simulink model "sampleModel2438_pp"  (R2018a)
settings: Solver=VariableStepAuto  StartTime=0.0  StopTime=10.0  RelTol=1e-3
undefined symbols (not defined in the file or in its folder): DiscIntNeverNeededParam, sigbuilder_block
libraries: simulink x299
(part 4 of 6)

== system sampleModel2438_pp/cfblk261 ==
  cfblk1 : Inport
  Action Port : ActionPort  ActionType=else
  cfblk10 : DiscreteIntegrator  SampleTime=-1  ICPrevOutput=DiscIntNeverNeededParam  ICPrevScaledInput=DiscIntNeverNeededParam
  cfblk12 : Delay
  cfblk3 : DiscreteFir
  cfblk4 : DiscreteFilter
  cfblk5 : UnitDelay  SampleTime=-1
  cfblk6 : simulink/Discrete/Transfer Fcn Real Zero  ZeroZ=0.75  ICPrevInput=0.0  DoSatur=off
      settings: SourceProductName=Simulink  SourceProductBaseCode=SL
  cfblk7 : DiscreteFilter
  cfblk8 : simulink/Continuous/PID Controller (2DOF)  Controller=PID  TimeDomain=Discrete-time  SampleTime=-1  IntegratorMethod=Forward Euler  FilterMethod=Forward Euler  Form=Parallel  UseFilter=on  ControllerParametersSource=internal  P=1  I=1  D=0  N=100  b=1  c=1  InitialConditionSource=internal  InitialConditionForIntegrator=0  InitialConditionForFilter=0  ExternalReset=none  LimitOutput=off  UpperSaturationLimit=inf  LowerSaturationLimit=-inf  LinearizeAsGain=off  AntiWindupMode=none  Kb=1  TrackingMode=off  Kt=1  PParamMin=[]  PParamMax=[]  IParamMin=[]  IParamMax=[]  DParamMin=[]  DParamMax=[]  NParamMin=[]  NParamMax=[]  bParamMin=[]  bParamMax=[]  cParamMin=[]  cParamMax=[]  KbParamMin=[]  KbParamMax=[]  KtParamMin=[]  KtParamMax=[]  POutMin=[]  POutMax=[]  IOutMin=[]  IOutMax=[]  DOutMin=[]  DOutMax=[]  NOutMin=[]  NOutMax=[]  bOutMin=[]  bOutMax=[]  cOutMin=[]  cOutMax=[]  KbOutMin=[]  KbOutMax=[]  KtOutMin=[]  KtOutMax=[]  IntegratorOutMin=[]  IntegratorOutMax=[]  FilterOutMin=[]  FilterOutMax=[]  SumOutMin=[]  SumOutMax=[]  Sum1OutMin=[]  Sum1OutMax=[]  Sum2OutMin=[]  Sum2OutMax=[]  Sum3OutMin=[]  Sum3OutMax=[]  SumI1OutMin=[]  SumI1OutMax=[]  SumI2OutMin=[]  SumI2OutMax=[]  SumI3OutMin=[]  SumI3OutMax=[]  SumDOutMin=[]  SumDOutMax=[]  SaturationOutMin=[]  SaturationOutMax=[]  IntegratorContinuousStateAttributes=''  IntegratorStateMustResolveToSignalObject=off  IntegratorRTWStateStorageClass=Auto  FilterContinuousStateAttributes=''  FilterStateMustResolveToSignalObject=off  FilterRTWStateStorageClass=Auto  DifferentiatorICPrevScaledInput=0  DifferentiatorOutMin=[]  DifferentiatorOutMax=[]  FilterDiffOutCoefMin=[]  FilterDiffOutCoefMax=[]  SumDenOutMin=[]  SumDenOutMax=[]  SumNumOutMin=[]  SumNumOutMax=[]  ReciprocalOutMin=[]  ReciprocalOutMax=[]  DivideOutMin=[]  DivideOutMax=[]  TunerSelectOption=Transfer Function Based (PID Tuner App)
  cfblk9 : DiscreteZeroPole  Poles=[0 0.5]  Gain=1  SampleTime=-1
  cyemi_{797..806} (10 alike) : DataTypeConversion  OutDataTypeStr=double
  cfblk2 : Outport
  cfblk11 : Outport  Port=2
  wires:
  cfblk5/1 -> cyemi_803/1, cyemi_806/1
  cfblk7/1 -> cfblk2/1
  cfblk1/1 -> cyemi_801/1, cyemi_804/1
  cfblk3/1 -> cfblk11/1
  cyemi_797/1 -> cfblk10/1
  cfblk6/1 -> cyemi_797/1
  cyemi_798/1 -> cfblk12/1
  cfblk10/1 -> cyemi_798/1
  cyemi_799/1 -> cfblk3/1
  cfblk4/1 -> cyemi_799/1
  cyemi_800/1 -> cfblk4/1
  cfblk9/1 -> cyemi_800/1
  cyemi_801/1 -> cfblk5/1
  cyemi_802/1 -> cfblk6/1
  cfblk8/1 -> cyemi_802/1
  cyemi_803/1 -> cfblk7/1
  cyemi_804/1 -> cfblk8/1
  cyemi_805/1 -> cfblk8/2
  cfblk12/1 -> cyemi_805/1
  cyemi_806/1 -> cfblk9/1

== system sampleModel2438_pp/cfblk262 ==
  cfblk1 : Inport
  Action Port : ActionPort  ActionType=then
  cfblk10 : Delay
  cfblk11 : Delay
  cfblk12 : Delay
  cfblk3 : simulink/Discrete/Transfer Fcn First Order  PoleZ=0.95  ICPrevOutput=0.0  DoSatur=off
      settings: SourceProductName=Simulink
  cfblk4 : simulink/Discrete/Transfer Fcn First Order  PoleZ=0.95  ICPrevOutput=0.0  DoSatur=off
      settings: SourceProductName=Simulink
  cfblk5 : simulink/Discrete/Transfer Fcn First Order  PoleZ=0.95  ICPrevOutput=0.0  DoSatur=off
      settings: SourceProductName=Simulink
  cfblk6 : If  SampleTime=1
  cfblk8 : Subsystem  TreatAsAtomicUnit=on
  cfblk9 : Subsystem  TreatAsAtomicUnit=on
  cyemi_{808..817,836..839} (14 alike) : DataTypeConversion  OutDataTypeStr=double
  cfblk2 : Outport
  cfblk7 : Outport  Port=2
  wires:
  cfblk9/1(cfblk2) -> cfblk7/1
  cfblk1/1 -> cyemi_813/1, cyemi_836/1
  cfblk3/1 -> cyemi_809/1, cyemi_810/1
  cfblk4/1 -> cfblk2/1, cyemi_808/1
  cfblk5/1 -> cyemi_814/1, cyemi_815/1, cyemi_838/1
  cfblk9/2(cfblk14) -> cyemi_812/1, cyemi_816/1
  cfblk6/1 -> cfblk8/Action
  cfblk6/2 -> cfblk9/Action
  cyemi_808/1 -> cfblk10/1
  cyemi_809/1 -> cfblk11/1
  cyemi_810/1 -> cfblk12/1
  cyemi_811/1 -> cfblk3/1
  cfblk8/1(cfblk2) -> cyemi_811/1
  cyemi_812/1 -> cfblk4/1
  cyemi_813/1 -> cfblk5/1
  cyemi_814/1 -> cfblk6/1
  cyemi_815/1 -> cfblk8/1(cfblk1)
  cyemi_816/1 -> cfblk8/2(cfblk14)
  cyemi_817/1 -> cfblk8/3(cfblk15)
  cfblk12/1 -> cyemi_817/1
  cyemi_836/1 -> cfblk9/1(cfblk1)
  cyemi_837/1 -> cfblk9/2(cfblk11)
  cfblk11/1 -> cyemi_837/1
  cyemi_838/1 -> cfblk9/3(cfblk12)
  cyemi_839/1 -> cfblk9/4(cfblk13)
  cfblk10/1 -> cyemi_839/1

== system sampleModel2438_pp/cfblk263 ==
  cfblk1 : Inport
  cfblk5 : Inport  Port=2
  cfblk6 : Inport  Port=3
  cfblk7 : Inport  Port=4
  Action Port : ActionPort  ActionType=else
  cfblk10 : Delay
  cfblk3 : Delay  ShowEnablePort=on
      settings: InputPortMap=u0,e6
  cfblk4 : Delay
  cyemi_{855..858} (4 alike) : DataTypeConversion  OutDataTypeStr=double
  cfblk2 : Outport
  cfblk8 : Outport  Port=2
  cfblk9 : Outport  Port=3
  wires:
  cfblk1/1 -> cfblk2/1
  cfblk6/1 -> cfblk9/1
  cfblk7/1 -> cfblk8/1
  cyemi_855/1 -> cfblk10/1
  cfblk4/1 -> cyemi_855/1
  cyemi_856/1 -> cfblk3/1
  cfblk5/1 -> cyemi_856/1
  cyemi_857/1 -> cfblk3/2
  cfblk10/1 -> cyemi_857/1
  cyemi_858/1 -> cfblk4/1
  cfblk3/1 -> cyemi_858/1

== system sampleModel2438_pp/cfblk264 ==
  cfblk1 : Inport
  cfblk6 : Inport  Port=2
  cfblk7 : Inport  Port=3
  Action Port : ActionPort  ActionType=then
  cfblk3 : simulink/Discrete/Tapped Delay  vinit=0.0  samptime=-1  NumDelays=1  DelayOrder=Oldest  includeCurrent=off
  cfblk4 : UnitDelay  SampleTime=-1
  cfblk5 : simulink/Discrete/Transfer Fcn Real Zero  ZeroZ=0.75  ICPrevInput=0.0  DoSatur=off
      settings: SourceProductName=Simulink  SourceProductBaseCode=SL
  cyemi_862 : DataTypeConversion  OutDataTypeStr=double
  cyemi_863 : DataTypeConversion  OutDataTypeStr=double
  cyemi_864 : DataTypeConversion  OutDataTypeStr=double
  cfblk2 : Outport
  wires:
  cfblk1/1 -> cfblk2/1
  cyemi_862/1 -> cfblk3/1
  cfblk7/1 -> cyemi_862/1
  cyemi_863/1 -> cfblk4/1
  cfblk5/1 -> cyemi_863/1
  cyemi_864/1 -> cfblk5/1
  cfblk3/1 -> cyemi_864/1

== system sampleModel2438_pp/cfblk265 ==
  cfblk1 : Inport
  cfblk6 : Inport  Port=2
  cfblk7 : Inport  Port=3
  cfblk8 : Inport  Port=4
  cfblk9 : Inport  Port=5
  Action Port : ActionPort  ActionType=else
  cfblk3 : DiscreteTransferFcn
  cfblk4 : DiscreteTransferFcn
  cfblk5 : DiscreteStateSpace  SampleTime=-1
  cyemi_870 : DataTypeConversion  OutDataTypeStr=double
  cyemi_871 : DataTypeConversion  OutDataTypeStr=double
  cyemi_872 : DataTypeConversion  OutDataTypeStr=double
  cfblk2 : Outport
  cfblk10 : Outport  Port=2
  wires:
  cfblk5/1 -> cfblk2/1
  cfblk9/1 -> cfblk10/1
  cyemi_870/1 -> cfblk3/1
  cfblk1/1 -> cyemi_870/1
  cyemi_871/1 -> cfblk4/1
  cfblk6/1 -> cyemi_871/1
  cyemi_872/1 -> cfblk5/1
  cfblk4/1 -> cyemi_872/1

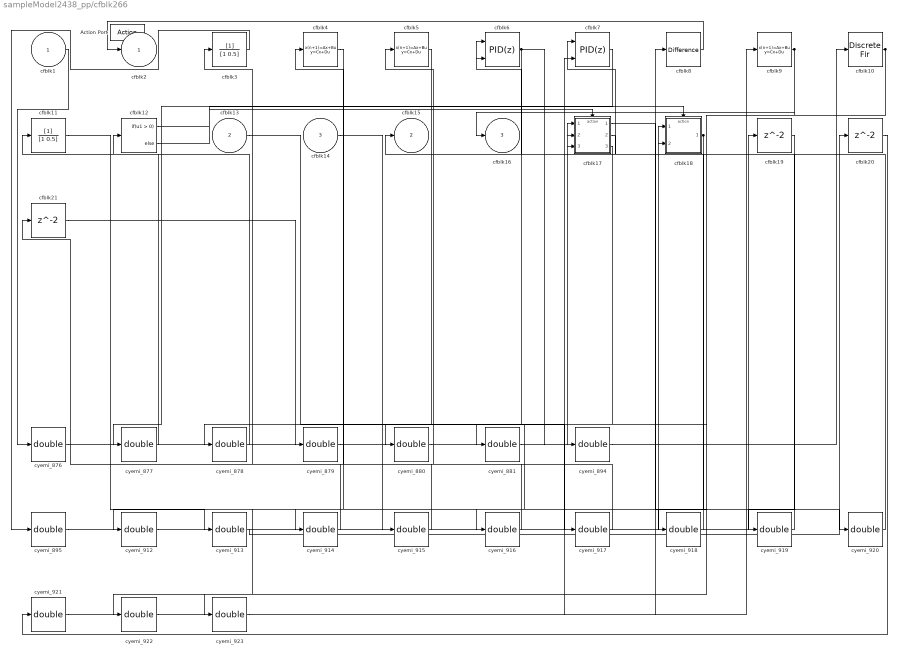
== system sampleModel2438_pp/cfblk266 ==
  cfblk1 : Inport
  cfblk13 : Inport  Port=2
  cfblk14 : Inport  Port=3
  Action Port : ActionPort  ActionType=then
  cfblk10 : DiscreteFir
  cfblk11 : DiscreteFilter
  cfblk12 : If  SampleTime=1
  cfblk17 : Subsystem  TreatAsAtomicUnit=on
  cfblk18 : Subsystem  TreatAsAtomicUnit=on
  cfblk19 : Delay
  cfblk20 : Delay
  cfblk21 : Delay
  cfblk3 : DiscreteFilter
  cfblk4 : DiscreteStateSpace  SampleTime=-1
  cfblk5 : DiscreteStateSpace  SampleTime=-1
  cfblk6 : simulink/Continuous/PID Controller (2DOF)  Controller=PID  TimeDomain=Discrete-time  SampleTime=-1  IntegratorMethod=Forward Euler  FilterMethod=Forward Euler  Form=Parallel  UseFilter=on  ControllerParametersSource=internal  P=1  I=1  D=0  N=100  b=1  c=1  InitialConditionSource=internal  InitialConditionForIntegrator=0  InitialConditionForFilter=0  ExternalReset=none  LimitOutput=off  UpperSaturationLimit=inf  LowerSaturationLimit=-inf  LinearizeAsGain=off  AntiWindupMode=none  Kb=1  TrackingMode=off  Kt=1  PParamMin=[]  PParamMax=[]  IParamMin=[]  IParamMax=[]  DParamMin=[]  DParamMax=[]  NParamMin=[]  NParamMax=[]  bParamMin=[]  bParamMax=[]  cParamMin=[]  cParamMax=[]  KbParamMin=[]  KbParamMax=[]  KtParamMin=[]  KtParamMax=[]  POutMin=[]  POutMax=[]  IOutMin=[]  IOutMax=[]  DOutMin=[]  DOutMax=[]  NOutMin=[]  NOutMax=[]  bOutMin=[]  bOutMax=[]  cOutMin=[]  cOutMax=[]  KbOutMin=[]  KbOutMax=[]  KtOutMin=[]  KtOutMax=[]  IntegratorOutMin=[]  IntegratorOutMax=[]  FilterOutMin=[]  FilterOutMax=[]  SumOutMin=[]  SumOutMax=[]  Sum1OutMin=[]  Sum1OutMax=[]  Sum2OutMin=[]  Sum2OutMax=[]  Sum3OutMin=[]  Sum3OutMax=[]  SumI1OutMin=[]  SumI1OutMax=[]  SumI2OutMin=[]  SumI2OutMax=[]  SumI3OutMin=[]  SumI3OutMax=[]  SumDOutMin=[]  SumDOutMax=[]  SaturationOutMin=[]  SaturationOutMax=[]  IntegratorContinuousStateAttributes=''  IntegratorStateMustResolveToSignalObject=off  IntegratorRTWStateStorageClass=Auto  FilterContinuousStateAttributes=''  FilterStateMustResolveToSignalObject=off  FilterRTWStateStorageClass=Auto  DifferentiatorICPrevScaledInput=0  DifferentiatorOutMin=[]  DifferentiatorOutMax=[]  FilterDiffOutCoefMin=[]  FilterDiffOutCoefMax=[]  SumDenOutMin=[]  SumDenOutMax=[]  SumNumOutMin=[]  SumNumOutMax=[]  ReciprocalOutMin=[]  ReciprocalOutMax=[]  DivideOutMin=[]  DivideOutMax=[]  TunerSelectOption=Transfer Function Based (PID Tuner App)
  cfblk7 : simulink/Continuous/PID Controller (2DOF)  Controller=PID  TimeDomain=Discrete-time  SampleTime=-1  IntegratorMethod=Forward Euler  FilterMethod=Forward Euler  Form=Parallel  UseFilter=on  ControllerParametersSource=internal  P=1  I=1  D=0  N=100  b=1  c=1  InitialConditionSource=internal  InitialConditionForIntegrator=0  InitialConditionForFilter=0  ExternalReset=none  LimitOutput=off  UpperSaturationLimit=inf  LowerSaturationLimit=-inf  LinearizeAsGain=off  AntiWindupMode=none  Kb=1  TrackingMode=off  Kt=1  PParamMin=[]  PParamMax=[]  IParamMin=[]  IParamMax=[]  DParamMin=[]  DParamMax=[]  NParamMin=[]  NParamMax=[]  bParamMin=[]  bParamMax=[]  cParamMin=[]  cParamMax=[]  KbParamMin=[]  KbParamMax=[]  KtParamMin=[]  KtParamMax=[]  POutMin=[]  POutMax=[]  IOutMin=[]  IOutMax=[]  DOutMin=[]  DOutMax=[]  NOutMin=[]  NOutMax=[]  bOutMin=[]  bOutMax=[]  cOutMin=[]  cOutMax=[]  KbOutMin=[]  KbOutMax=[]  KtOutMin=[]  KtOutMax=[]  IntegratorOutMin=[]  IntegratorOutMax=[]  FilterOutMin=[]  FilterOutMax=[]  SumOutMin=[]  SumOutMax=[]  Sum1OutMin=[]  Sum1OutMax=[]  Sum2OutMin=[]  Sum2OutMax=[]  Sum3OutMin=[]  Sum3OutMax=[]  SumI1OutMin=[]  SumI1OutMax=[]  SumI2OutMin=[]  SumI2OutMax=[]  SumI3OutMin=[]  SumI3OutMax=[]  SumDOutMin=[]  SumDOutMax=[]  SaturationOutMin=[]  SaturationOutMax=[]  IntegratorContinuousStateAttributes=''  IntegratorStateMustResolveToSignalObject=off  IntegratorRTWStateStorageClass=Auto  FilterContinuousStateAttributes=''  FilterStateMustResolveToSignalObject=off  FilterRTWStateStorageClass=Auto  DifferentiatorICPrevScaledInput=0  DifferentiatorOutMin=[]  DifferentiatorOutMax=[]  FilterDiffOutCoefMin=[]  FilterDiffOutCoefMax=[]  SumDenOutMin=[]  SumDenOutMax=[]  SumNumOutMin=[]  SumNumOutMax=[]  ReciprocalOutMin=[]  ReciprocalOutMax=[]  DivideOutMin=[]  DivideOutMax=[]  TunerSelectOption=Transfer Function Based (PID Tuner App)
  cfblk8 : simulink/Discrete/Difference  ICPrevInput=0.0  OutMin=[]  OutMax=[]  OutDataTypeStr=Inherit: Inherit via back propagation  OutDataType=fixdt(1, 16)  OutScaling=2^-10  DoSatur=off
  cfblk9 : DiscreteStateSpace  SampleTime=-1
  cyemi_{876..881,894..895,912..923} (20 alike) : DataTypeConversion  OutDataTypeStr=double
  cfblk2 : Outport
  cfblk15 : Outport  Port=2
  cfblk16 : Outport  Port=3
  wires:
  cfblk6/1 -> cyemi_880/1, cyemi_894/1
  cfblk17/2(cfblk11) -> cfblk15/1
  cfblk8/1 -> cfblk2/1
  cfblk10/1 -> cyemi_881/1, cyemi_918/1
  cfblk18/1(cfblk2) -> cyemi_912/1, cyemi_923/1
  cfblk9/1 -> cfblk16/1, cyemi_922/1
  cfblk12/1 -> cfblk17/Action
  cfblk12/2 -> cfblk18/Action
  cyemi_876/1 -> cfblk10/1
  cfblk1/1 -> cyemi_876/1
  cyemi_877/1 -> cfblk11/1
  cfblk7/1 -> cyemi_877/1
  cyemi_878/1 -> cfblk12/1
  cfblk5/1 -> cyemi_878/1
  cyemi_879/1 -> cfblk17/1(cfblk1)
  cfblk21/1 -> cyemi_879/1
  cyemi_880/1 -> cfblk17/2(cfblk9)
  cyemi_881/1 -> cfblk17/3(cfblk10)
  cyemi_894/1 -> cfblk18/1(cfblk1)
  cyemi_895/1 -> cfblk18/2(cfblk14)
  cfblk3/1 -> cyemi_895/1
  cyemi_912/1 -> cfblk19/1
  cyemi_913/1 -> cfblk20/1
  cfblk11/1 -> cyemi_913/1
  cyemi_914/1 -> cfblk21/1
  cfblk4/1 -> cyemi_914/1
  cyemi_915/1 -> cfblk3/1
  cfblk14/1 -> cyemi_915/1
  cyemi_916/1 -> cfblk4/1
  cfblk17/3(cfblk12) -> cyemi_916/1
  cyemi_917/1 -> cfblk5/1
  cfblk13/1 -> cyemi_917/1
  cyemi_918/1 -> cfblk6/1
  cyemi_919/1 -> cfblk6/2
  cfblk19/1 -> cyemi_919/1
  cyemi_920/1 -> cfblk7/1
  cfblk17/1(cfblk2) -> cyemi_920/1
  cyemi_921/1 -> cfblk7/2
  cfblk20/1 -> cyemi_921/1
  cyemi_922/1 -> cfblk8/1
  cyemi_923/1 -> cfblk9/1

== system sampleModel2438_pp/cfblk267 ==
  cfblk1 : Inport
  cfblk10 : Inport  Port=2
  cfblk11 : Inport  Port=3
  cfblk12 : Inport  Port=4
  Action Port : ActionPort  ActionType=else
  cfblk15 : Delay
  cfblk3 : simulink/Discrete/Difference  ICPrevInput=0.0  OutMin=[]  OutMax=[]  OutDataTypeStr=Inherit: Inherit via back propagation  OutDataType=fixdt(1, 16)  OutScaling=2^-10  DoSatur=off
  cfblk4 : DiscreteTransferFcn
  cfblk5 : simulink/Discrete/Transfer Fcn Real Zero  ZeroZ=0.75  ICPrevInput=0.0  DoSatur=off
      settings: SourceProductName=Simulink  SourceProductBaseCode=SL
  cfblk6 : DiscreteIntegrator  SampleTime=-1  ICPrevOutput=DiscIntNeverNeededParam  ICPrevScaledInput=DiscIntNeverNeededParam
  cfblk7 : simulink/Continuous/PID Controller (2DOF)  Controller=PID  TimeDomain=Discrete-time  SampleTime=-1  IntegratorMethod=Forward Euler  FilterMethod=Forward Euler  Form=Parallel  UseFilter=on  ControllerParametersSource=internal  P=1  I=1  D=0  N=100  b=1  c=1  InitialConditionSource=internal  InitialConditionForIntegrator=0  InitialConditionForFilter=0  ExternalReset=none  LimitOutput=off  UpperSaturationLimit=inf  LowerSaturationLimit=-inf  LinearizeAsGain=off  AntiWindupMode=none  Kb=1  TrackingMode=off  Kt=1  PParamMin=[]  PParamMax=[]  IParamMin=[]  IParamMax=[]  DParamMin=[]  DParamMax=[]  NParamMin=[]  NParamMax=[]  bParamMin=[]  bParamMax=[]  cParamMin=[]  cParamMax=[]  KbParamMin=[]  KbParamMax=[]  KtParamMin=[]  KtParamMax=[]  POutMin=[]  POutMax=[]  IOutMin=[]  IOutMax=[]  DOutMin=[]  DOutMax=[]  NOutMin=[]  NOutMax=[]  bOutMin=[]  bOutMax=[]  cOutMin=[]  cOutMax=[]  KbOutMin=[]  KbOutMax=[]  KtOutMin=[]  KtOutMax=[]  IntegratorOutMin=[]  IntegratorOutMax=[]  FilterOutMin=[]  FilterOutMax=[]  SumOutMin=[]  SumOutMax=[]  Sum1OutMin=[]  Sum1OutMax=[]  Sum2OutMin=[]  Sum2OutMax=[]  Sum3OutMin=[]  Sum3OutMax=[]  SumI1OutMin=[]  SumI1OutMax=[]  SumI2OutMin=[]  SumI2OutMax=[]  SumI3OutMin=[]  SumI3OutMax=[]  SumDOutMin=[]  SumDOutMax=[]  SaturationOutMin=[]  SaturationOutMax=[]  IntegratorContinuousStateAttributes=''  IntegratorStateMustResolveToSignalObject=off  IntegratorRTWStateStorageClass=Auto  FilterContinuousStateAttributes=''  FilterStateMustResolveToSignalObject=off  FilterRTWStateStorageClass=Auto  DifferentiatorICPrevScaledInput=0  DifferentiatorOutMin=[]  DifferentiatorOutMax=[]  FilterDiffOutCoefMin=[]  FilterDiffOutCoefMax=[]  SumDenOutMin=[]  SumDenOutMax=[]  SumNumOutMin=[]  SumNumOutMax=[]  ReciprocalOutMin=[]  ReciprocalOutMax=[]  DivideOutMin=[]  DivideOutMax=[]  TunerSelectOption=Transfer Function Based (PID Tuner App)
  cfblk8 : simulink/Discrete/Transfer Fcn Real Zero  ZeroZ=0.75  ICPrevInput=0.0  DoSatur=off
      settings: SourceProductName=Simulink  SourceProductBaseCode=SL
  cfblk9 : DiscreteStateSpace  SampleTime=-1
  cyemi_{928..936} (9 alike) : DataTypeConversion  OutDataTypeStr=double
  cfblk2 : Outport
  cfblk13 : Outport  Port=2
  cfblk14 : Outport  Port=3
  wires:
  cfblk8/1 -> cfblk14/1
  cfblk6/1 -> cfblk13/1
  cfblk1/1 -> cfblk2/1
  cyemi_928/1 -> cfblk15/1
  cfblk9/1 -> cyemi_928/1
  cyemi_929/1 -> cfblk3/1
  cfblk4/1 -> cyemi_929/1
  cyemi_930/1 -> cfblk4/1
  cfblk12/1 -> cyemi_930/1
  cyemi_931/1 -> cfblk5/1
  cfblk15/1 -> cyemi_931/1
  cyemi_932/1 -> cfblk6/1
  cfblk7/1 -> cyemi_932/1
  cyemi_933/1 -> cfblk7/1
  cfblk3/1 -> cyemi_933/1
  cyemi_934/1 -> cfblk7/2
  cfblk10/1 -> cyemi_934/1
  cyemi_935/1 -> cfblk8/1
  cfblk11/1 -> cyemi_935/1
  cyemi_936/1 -> cfblk9/1
  cfblk5/1 -> cyemi_936/1

== system sampleModel2438_pp/cfblk268 ==
  cfblk1 : Inport
  cfblk7 : Inport  Port=2
  Action Port : ActionPort  ActionType=then
  cfblk3 : Delay  DelayLengthSource=Input port
      settings: InputPortMap=u0,p1
  cfblk4 : simulink/Discrete/Transfer Fcn First Order  PoleZ=0.95  ICPrevOutput=0.0  DoSatur=off
      settings: SourceProductName=Simulink
  cfblk5 : DiscreteZeroPole  Poles=[0 0.5]  Gain=1  SampleTime=-1
  cfblk6 : simulink/Continuous/PID Controller (2DOF)  Controller=PID  TimeDomain=Discrete-time  SampleTime=-1  IntegratorMethod=Forward Euler  FilterMethod=Forward Euler  Form=Parallel  UseFilter=on  ControllerParametersSource=internal  P=1  I=1  D=0  N=100  b=1  c=1  InitialConditionSource=internal  InitialConditionForIntegrator=0  InitialConditionForFilter=0  ExternalReset=none  LimitOutput=off  UpperSaturationLimit=inf  LowerSaturationLimit=-inf  LinearizeAsGain=off  AntiWindupMode=none  Kb=1  TrackingMode=off  Kt=1  PParamMin=[]  PParamMax=[]  IParamMin=[]  IParamMax=[]  DParamMin=[]  DParamMax=[]  NParamMin=[]  NParamMax=[]  bParamMin=[]  bParamMax=[]  cParamMin=[]  cParamMax=[]  KbParamMin=[]  KbParamMax=[]  KtParamMin=[]  KtParamMax=[]  POutMin=[]  POutMax=[]  IOutMin=[]  IOutMax=[]  DOutMin=[]  DOutMax=[]  NOutMin=[]  NOutMax=[]  bOutMin=[]  bOutMax=[]  cOutMin=[]  cOutMax=[]  KbOutMin=[]  KbOutMax=[]  KtOutMin=[]  KtOutMax=[]  IntegratorOutMin=[]  IntegratorOutMax=[]  FilterOutMin=[]  FilterOutMax=[]  SumOutMin=[]  SumOutMax=[]  Sum1OutMin=[]  Sum1OutMax=[]  Sum2OutMin=[]  Sum2OutMax=[]  Sum3OutMin=[]  Sum3OutMax=[]  SumI1OutMin=[]  SumI1OutMax=[]  SumI2OutMin=[]  SumI2OutMax=[]  SumI3OutMin=[]  SumI3OutMax=[]  SumDOutMin=[]  SumDOutMax=[]  SaturationOutMin=[]  SaturationOutMax=[]  IntegratorContinuousStateAttributes=''  IntegratorStateMustResolveToSignalObject=off  IntegratorRTWStateStorageClass=Auto  FilterContinuousStateAttributes=''  FilterStateMustResolveToSignalObject=off  FilterRTWStateStorageClass=Auto  DifferentiatorICPrevScaledInput=0  DifferentiatorOutMin=[]  DifferentiatorOutMax=[]  FilterDiffOutCoefMin=[]  FilterDiffOutCoefMax=[]  SumDenOutMin=[]  SumDenOutMax=[]  SumNumOutMin=[]  SumNumOutMax=[]  ReciprocalOutMin=[]  ReciprocalOutMax=[]  DivideOutMin=[]  DivideOutMax=[]  TunerSelectOption=Transfer Function Based (PID Tuner App)
  cfblk9 : Delay
  cyemi_{939,941..942,944..945} (5 alike) : DataTypeConversion  OutDataTypeStr=double
  cyemi_940 : DataTypeConversion  OutDataTypeStr=uint32
  cyemi_943 : DataTypeConversion  OutDataTypeStr=uint32
  cfblk2 : Outport
  cfblk8 : Outport  Port=2
  wires:
  cfblk1/1 -> cyemi_940/1, cyemi_943/1
  cfblk6/1 -> cfblk2/1
  cfblk4/1 -> cfblk8/1, cyemi_945/1
  cyemi_939/1 -> cfblk3/1
  cfblk9/1 -> cyemi_939/1
  cyemi_940/1 -> cfblk3/2
  cyemi_941/1 -> cfblk4/1
  cfblk3/1 -> cyemi_941/1
  cyemi_942/1 -> cfblk5/1
  cfblk7/1 -> cyemi_942/1
  cyemi_943/1 -> cfblk6/1
  cyemi_944/1 -> cfblk6/2
  cfblk5/1 -> cyemi_944/1
  cyemi_945/1 -> cfblk9/1

== system sampleModel2438_pp/cfblk269 ==
  cfblk1 : Inport
  cfblk10 : Inport  Port=2
  Action Port : ActionPort  ActionType=else
  cfblk11 : Delay
  cfblk3 : simulink/Continuous/PID Controller  Controller=PID  TimeDomain=Discrete-time  SampleTime=-1  IntegratorMethod=Forward Euler  FilterMethod=Forward Euler  Form=Parallel  UseFilter=on  ControllerParametersSource=internal  P=1  I=1  D=0  N=100  InitialConditionSource=internal  InitialConditionForIntegrator=0  InitialConditionForFilter=0  ExternalReset=none  LimitOutput=off  UpperSaturationLimit=inf  LowerSaturationLimit=-inf  LinearizeAsGain=off  AntiWindupMode=none  Kb=1  TrackingMode=off  Kt=1  PParamMin=[]  PParamMax=[]  IParamMin=[]  IParamMax=[]  DParamMin=[]  DParamMax=[]  NParamMin=[]  NParamMax=[]  KbParamMin=[]  KbParamMax=[]  KtParamMin=[]  KtParamMax=[]  POutMin=[]  POutMax=[]  IOutMin=[]  IOutMax=[]  DOutMin=[]  DOutMax=[]  NOutMin=[]  NOutMax=[]  KbOutMin=[]  KbOutMax=[]  KtOutMin=[]  KtOutMax=[]  IntegratorOutMin=[]  IntegratorOutMax=[]  FilterOutMin=[]  FilterOutMax=[]  SumOutMin=[]  SumOutMax=[]  SumI1OutMin=[]  SumI1OutMax=[]  SumI2OutMin=[]  SumI2OutMax=[]  SumI3OutMin=[]  SumI3OutMax=[]  SumDOutMin=[]  SumDOutMax=[]  SaturationOutMin=[]  SaturationOutMax=[]  IntegratorContinuousStateAttributes=''  IntegratorStateMustResolveToSignalObject=off  IntegratorRTWStateStorageClass=Auto  FilterContinuousStateAttributes=''  FilterStateMustResolveToSignalObject=off  FilterRTWStateStorageClass=Auto  DifferentiatorICPrevScaledInput=0  DifferentiatorOutMin=[]  DifferentiatorOutMax=[]  FilterDiffOutCoefMin=[]  FilterDiffOutCoefMax=[]  SumDenOutMin=[]  SumDenOutMax=[]  SumNumOutMin=[]  SumNumOutMax=[]  ReciprocalOutMin=[]  ReciprocalOutMax=[]  DivideOutMin=[]  DivideOutMax=[]  TunerSelectOption=Transfer Function Based (PID Tuner App)
  cfblk4 : simulink/Continuous/PID Controller  Controller=PID  TimeDomain=Discrete-time  SampleTime=-1  IntegratorMethod=Forward Euler  FilterMethod=Forward Euler  Form=Parallel  UseFilter=on  ControllerParametersSource=internal  P=1  I=1  D=0  N=100  InitialConditionSource=internal  InitialConditionForIntegrator=0  InitialConditionForFilter=0  ExternalReset=none  LimitOutput=off  UpperSaturationLimit=inf  LowerSaturationLimit=-inf  LinearizeAsGain=off  AntiWindupMode=none  Kb=1  TrackingMode=off  Kt=1  PParamMin=[]  PParamMax=[]  IParamMin=[]  IParamMax=[]  DParamMin=[]  DParamMax=[]  NParamMin=[]  NParamMax=[]  KbParamMin=[]  KbParamMax=[]  KtParamMin=[]  KtParamMax=[]  POutMin=[]  POutMax=[]  IOutMin=[]  IOutMax=[]  DOutMin=[]  DOutMax=[]  NOutMin=[]  NOutMax=[]  KbOutMin=[]  KbOutMax=[]  KtOutMin=[]  KtOutMax=[]  IntegratorOutMin=[]  IntegratorOutMax=[]  FilterOutMin=[]  FilterOutMax=[]  SumOutMin=[]  SumOutMax=[]  SumI1OutMin=[]  SumI1OutMax=[]  SumI2OutMin=[]  SumI2OutMax=[]  SumI3OutMin=[]  SumI3OutMax=[]  SumDOutMin=[]  SumDOutMax=[]  SaturationOutMin=[]  SaturationOutMax=[]  IntegratorContinuousStateAttributes=''  IntegratorStateMustResolveToSignalObject=off  IntegratorRTWStateStorageClass=Auto  FilterContinuousStateAttributes=''  FilterStateMustResolveToSignalObject=off  FilterRTWStateStorageClass=Auto  DifferentiatorICPrevScaledInput=0  DifferentiatorOutMin=[]  DifferentiatorOutMax=[]  FilterDiffOutCoefMin=[]  FilterDiffOutCoefMax=[]  SumDenOutMin=[]  SumDenOutMax=[]  SumNumOutMin=[]  SumNumOutMax=[]  ReciprocalOutMin=[]  ReciprocalOutMax=[]  DivideOutMin=[]  DivideOutMax=[]  TunerSelectOption=Transfer Function Based (PID Tuner App)
  cfblk5 : DiscreteIntegrator  SampleTime=-1  ICPrevOutput=DiscIntNeverNeededParam  ICPrevScaledInput=DiscIntNeverNeededParam
  cfblk6 : simulink/Discrete/Transfer Fcn First Order  PoleZ=0.95  ICPrevOutput=0.0  DoSatur=off
      settings: SourceProductName=Simulink
  cfblk7 : UnitDelay  SampleTime=-1
  cfblk8 : DiscreteFilter
  cfblk9 : DiscreteStateSpace  SampleTime=-1
  cyemi_{948..955} (8 alike) : DataTypeConversion  OutDataTypeStr=double
  cfblk2 : Outport
  wires:
  cfblk3/1 -> cfblk2/1
  cyemi_948/1 -> cfblk11/1
  cfblk7/1 -> cyemi_948/1
  cyemi_949/1 -> cfblk3/1
  cfblk8/1 -> cyemi_949/1
  cyemi_950/1 -> cfblk4/1
  cfblk11/1 -> cyemi_950/1
  cyemi_951/1 -> cfblk5/1
  cfblk1/1 -> cyemi_951/1
  cyemi_952/1 -> cfblk6/1
  cfblk10/1 -> cyemi_952/1
  cyemi_953/1 -> cfblk7/1
  cfblk9/1 -> cyemi_953/1
  cyemi_954/1 -> cfblk8/1
  cfblk6/1 -> cyemi_954/1
  cyemi_955/1 -> cfblk9/1
  cfblk4/1 -> cyemi_955/1

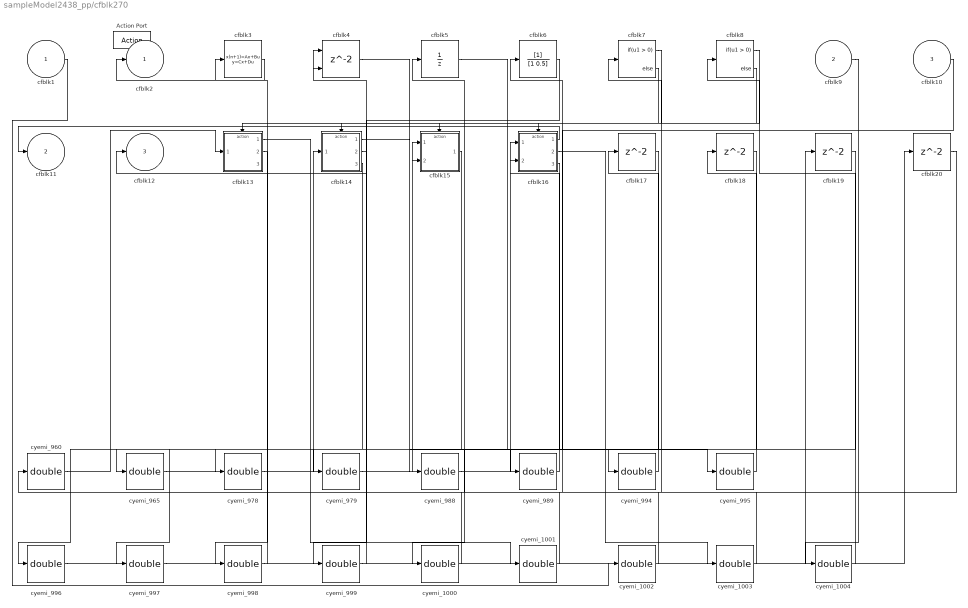
== system sampleModel2438_pp/cfblk270 ==
  cfblk1 : Inport
  cfblk9 : Inport  Port=2
  cfblk10 : Inport  Port=3
  Action Port : ActionPort  ActionType=then
  cfblk13 : Subsystem  TreatAsAtomicUnit=on
  cfblk14 : Subsystem  TreatAsAtomicUnit=on
  cfblk15 : Subsystem  TreatAsAtomicUnit=on
  cfblk16 : Subsystem  TreatAsAtomicUnit=on
  cfblk{17..20} (4 alike) : Delay
  cfblk3 : DiscreteStateSpace  SampleTime=-1
  cfblk4 : Delay  ShowEnablePort=on
      settings: InputPortMap=u0,e6
  cfblk5 : UnitDelay  SampleTime=-1
  cfblk6 : DiscreteFilter
  cfblk7 : If  SampleTime=1
  cfblk8 : If  SampleTime=1
  cyemi_{960,965,978..979,988..989,994..1004} (17 alike) : DataTypeConversion  OutDataTypeStr=double
  cfblk2 : Outport
  cfblk11 : Outport  Port=2
  cfblk12 : Outport  Port=3
  wires:
  cfblk16/1(cfblk2) -> cfblk11/1
  cfblk14/2(cfblk12) -> cfblk12/1
  cfblk3/1 -> cfblk2/1
  cfblk7/1 -> cfblk13/Action
  cfblk7/2 -> cfblk14/Action
  cfblk8/1 -> cfblk15/Action
  cfblk8/2 -> cfblk16/Action
  cyemi_960/1 -> cfblk13/1(cfblk1)
  cfblk20/1 -> cyemi_960/1
  cyemi_965/1 -> cfblk14/1(cfblk1)
  cfblk13/2(cfblk6) -> cyemi_965/1
  cyemi_978/1 -> cfblk15/1(cfblk1)
  cfblk18/1 -> cyemi_978/1
  cyemi_979/1 -> cfblk15/2(cfblk9)
  cfblk10/1 -> cyemi_979/1
  cyemi_988/1 -> cfblk16/1(cfblk1)
  cfblk4/1 -> cyemi_988/1
  cyemi_989/1 -> cfblk16/2(cfblk7)
  cfblk19/1 -> cyemi_989/1
  cyemi_994/1 -> cfblk17/1
  cfblk5/1 -> cyemi_994/1
  cyemi_995/1 -> cfblk18/1
  cfblk14/1(cfblk2) -> cyemi_995/1
  cyemi_996/1 -> cfblk19/1
  cfblk15/1(cfblk2) -> cyemi_996/1
  cyemi_997/1 -> cfblk20/1
  cfblk14/3(cfblk13) -> cyemi_997/1
  cyemi_998/1 -> cfblk3/1
  cfblk16/3(cfblk9) -> cyemi_998/1
  cyemi_999/1 -> cfblk4/1
  cfblk6/1 -> cyemi_999/1
  cyemi_1000/1 -> cfblk4/2
  cfblk17/1 -> cyemi_1000/1
  cyemi_1001/1 -> cfblk5/1
  cfblk13/1(cfblk2) -> cyemi_1001/1
  cyemi_1002/1 -> cfblk6/1
  cfblk1/1 -> cyemi_1002/1
  cyemi_1003/1 -> cfblk7/1
  cfblk16/2(cfblk8) -> cyemi_1003/1
  cyemi_1004/1 -> cfblk8/1
  cfblk9/1 -> cyemi_1004/1

== system sampleModel2438_pp/cfblk271 ==
  cfblk1 : Inport
  cfblk8 : Inport  Port=2
  cfblk9 : Inport  Port=3
  Action Port : ActionPort  ActionType=else
  cfblk3 : DiscreteTransferFcn
  cfblk4 : DiscreteFilter
  cfblk5 : Delay  ShowEnablePort=on
      settings: InputPortMap=u0,e6
  cfblk6 : simulink/Discrete/Transfer Fcn First Order  PoleZ=0.95  ICPrevOutput=0.0  DoSatur=off
      settings: SourceProductName=Simulink
  cfblk7 : DiscreteTransferFcn
  cyemi_{1008..1013} (6 alike) : DataTypeConversion  OutDataTypeStr=double
  cfblk2 : Outport
  wires:
  cfblk1/1 -> cfblk2/1
  cyemi_1008/1 -> cfblk3/1
  cfblk5/1 -> cyemi_1008/1
  cyemi_1009/1 -> cfblk4/1
  cfblk7/1 -> cyemi_1009/1
  cyemi_1010/1 -> cfblk5/1
  cfblk9/1 -> cyemi_1010/1
  cyemi_1011/1 -> cfblk5/2
  cfblk6/1 -> cyemi_1011/1
  cyemi_1012/1 -> cfblk6/1
  cfblk4/1 -> cyemi_1012/1
  cyemi_1013/1 -> cfblk7/1
  cfblk8/1 -> cyemi_1013/1

== system sampleModel2438_pp/cfblk272 ==
  cfblk1 : Inport
  cfblk10 : Inport  Port=2
  Action Port : ActionPort  ActionType=then
  cfblk11 : Delay
  cfblk12 : Delay
  cfblk3 : Delay  DelayLengthSource=Input port
      settings: InputPortMap=u0,p1
  cfblk4 : DiscreteFilter
  cfblk5 : UnitDelay  SampleTime=-1
  cfblk6 : DiscreteIntegrator  SampleTime=-1  ICPrevOutput=DiscIntNeverNeededParam  ICPrevScaledInput=DiscIntNeverNeededParam
  cfblk7 : DiscreteFir
  cfblk8 : DiscreteFilter
  cfblk9 : simulink/Continuous/PID Controller  Controller=PID  TimeDomain=Discrete-time  SampleTime=-1  IntegratorMethod=Forward Euler  FilterMethod=Forward Euler  Form=Parallel  UseFilter=on  ControllerParametersSource=internal  P=1  I=1  D=0  N=100  InitialConditionSource=internal  InitialConditionForIntegrator=0  InitialConditionForFilter=0  ExternalReset=none  LimitOutput=off  UpperSaturationLimit=inf  LowerSaturationLimit=-inf  LinearizeAsGain=off  AntiWindupMode=none  Kb=1  TrackingMode=off  Kt=1  PParamMin=[]  PParamMax=[]  IParamMin=[]  IParamMax=[]  DParamMin=[]  DParamMax=[]  NParamMin=[]  NParamMax=[]  KbParamMin=[]  KbParamMax=[]  KtParamMin=[]  KtParamMax=[]  POutMin=[]  POutMax=[]  IOutMin=[]  IOutMax=[]  DOutMin=[]  DOutMax=[]  NOutMin=[]  NOutMax=[]  KbOutMin=[]  KbOutMax=[]  KtOutMin=[]  KtOutMax=[]  IntegratorOutMin=[]  IntegratorOutMax=[]  FilterOutMin=[]  FilterOutMax=[]  SumOutMin=[]  SumOutMax=[]  SumI1OutMin=[]  SumI1OutMax=[]  SumI2OutMin=[]  SumI2OutMax=[]  SumI3OutMin=[]  SumI3OutMax=[]  SumDOutMin=[]  SumDOutMax=[]  SaturationOutMin=[]  SaturationOutMax=[]  IntegratorContinuousStateAttributes=''  IntegratorStateMustResolveToSignalObject=off  IntegratorRTWStateStorageClass=Auto  FilterContinuousStateAttributes=''  FilterStateMustResolveToSignalObject=off  FilterRTWStateStorageClass=Auto  DifferentiatorICPrevScaledInput=0  DifferentiatorOutMin=[]  DifferentiatorOutMax=[]  FilterDiffOutCoefMin=[]  FilterDiffOutCoefMax=[]  SumDenOutMin=[]  SumDenOutMax=[]  SumNumOutMin=[]  SumNumOutMax=[]  ReciprocalOutMin=[]  ReciprocalOutMax=[]  DivideOutMin=[]  DivideOutMax=[]  TunerSelectOption=Transfer Function Based (PID Tuner App)
  cyemi_{1016..1025} (10 alike) : DataTypeConversion  OutDataTypeStr=double
  cfblk2 : Outport
  wires:
  cfblk10/1 -> cfblk2/1
  cyemi_1016/1 -> cfblk11/1
  cfblk5/1 -> cyemi_1016/1
  cyemi_1017/1 -> cfblk12/1
  cfblk6/1 -> cyemi_1017/1
  cyemi_1018/1 -> cfblk3/1
  cfblk9/1 -> cyemi_1018/1
  cyemi_1019/1 -> cfblk3/2
  cfblk11/1 -> cyemi_1019/1
  cyemi_1020/1 -> cfblk4/1
  cfblk12/1 -> cyemi_1020/1
  cyemi_1021/1 -> cfblk5/1
  cfblk7/1 -> cyemi_1021/1
  cyemi_1022/1 -> cfblk6/1
  cfblk4/1 -> cyemi_1022/1
  cyemi_1023/1 -> cfblk7/1
  cfblk3/1 -> cyemi_1023/1
  cyemi_1024/1 -> cfblk8/1
  cfblk1/1 -> cyemi_1024/1
  cyemi_1025/1 -> cfblk9/1
  cfblk8/1 -> cyemi_1025/1

== system sampleModel2438_pp/cfblk273 ==
  cfblk1 : Inport
  cfblk9 : Inport  Port=2
  cfblk10 : Inport  Port=3
  Action Port : ActionPort  ActionType=else
  cfblk11 : Delay
  cfblk3 : DiscreteStateSpace  SampleTime=-1
  cfblk4 : simulink/Discrete/Transfer Fcn Real Zero  ZeroZ=0.75  ICPrevInput=0.0  DoSatur=off
      settings: SourceProductName=Simulink  SourceProductBaseCode=SL
  cfblk5 : Delay  DelayLengthSource=Input port
      settings: InputPortMap=u0,p1
  cfblk6 : simulink/Discrete/Transfer Fcn Real Zero  ZeroZ=0.75  ICPrevInput=0.0  DoSatur=off
      settings: SourceProductName=Simulink  SourceProductBaseCode=SL
  cfblk7 : DiscreteStateSpace  SampleTime=-1
  cfblk8 : DiscreteStateSpace  SampleTime=-1
  cyemi_{1029..1036} (8 alike) : DataTypeConversion  OutDataTypeStr=double
  cfblk2 : Outport
  wires:
  cfblk1/1 -> cfblk2/1
  cyemi_1029/1 -> cfblk11/1
  cfblk6/1 -> cyemi_1029/1
  cyemi_1030/1 -> cfblk3/1
  cfblk9/1 -> cyemi_1030/1
  cyemi_1031/1 -> cfblk4/1
  cfblk11/1 -> cyemi_1031/1
  cyemi_1032/1 -> cfblk5/1
  cfblk8/1 -> cyemi_1032/1
  cyemi_1033/1 -> cfblk5/2
  cfblk3/1 -> cyemi_1033/1
  cyemi_1034/1 -> cfblk6/1
  cfblk4/1 -> cyemi_1034/1
  cyemi_1035/1 -> cfblk7/1
  cfblk5/1 -> cyemi_1035/1
  cyemi_1036/1 -> cfblk8/1
  cfblk10/1 -> cyemi_1036/1

== system sampleModel2438_pp/cfblk232/cfblk10 ==
  cfblk1 : Inport
  cfblk8 : Inport  Port=2
  cfblk9 : Inport  Port=3
  Action Port : ActionPort  ActionType=else
  cfblk11 : Delay
  cfblk3 : simulink/Discrete/Transfer Fcn Real Zero  ZeroZ=0.75  ICPrevInput=0.0  DoSatur=off
      settings: SourceProductName=Simulink  SourceProductBaseCode=SL
  cfblk4 : simulink/Discrete/Transfer Fcn First Order  PoleZ=0.95  ICPrevOutput=0.0  DoSatur=off
      settings: SourceProductName=Simulink
  cfblk5 : simulink/Discrete/Difference  ICPrevInput=0.0  OutMin=[]  OutMax=[]  OutDataTypeStr=Inherit: Inherit via back propagation  OutDataType=fixdt(1, 16)  OutScaling=2^-10  DoSatur=off
  cfblk6 : simulink/Discrete/Transfer Fcn Lead or Lag  PoleZ=0.95  ZeroZ=0.75  ICPrevOutput=0.0  ICPrevInput=0.0  DoSatur=off
      settings: SourceProductName=Simulink  SourceProductBaseCode=SL
  cfblk7 : Delay
  cyemi_{88..93} (6 alike) : DataTypeConversion  OutDataTypeStr=double
  cfblk2 : Outport
  cfblk10 : Outport  Port=2
  wires:
  cfblk9/1 -> cfblk10/1
  cfblk1/1 -> cfblk2/1
  cyemi_88/1 -> cfblk11/1
  cfblk6/1 -> cyemi_88/1
  cyemi_89/1 -> cfblk3/1
  cfblk11/1 -> cyemi_89/1
  cyemi_90/1 -> cfblk4/1
  cfblk5/1 -> cyemi_90/1
  cyemi_91/1 -> cfblk5/1
  cfblk7/1 -> cyemi_91/1
  cyemi_92/1 -> cfblk6/1
  cfblk4/1 -> cyemi_92/1
  cyemi_93/1 -> cfblk7/1
  cfblk3/1 -> cyemi_93/1

== system sampleModel2438_pp/cfblk232/cfblk9 ==
  cfblk1 : Inport
  cfblk9 : Inport  Port=2
  cfblk10 : Inport  Port=3
  Action Port : ActionPort  ActionType=then
  cfblk3 : simulink/Discrete/Transfer Fcn Real Zero  ZeroZ=0.75  ICPrevInput=0.0  DoSatur=off
      settings: SourceProductName=Simulink  SourceProductBaseCode=SL
  cfblk4 : simulink/Discrete/Transfer Fcn First Order  PoleZ=0.95  ICPrevOutput=0.0  DoSatur=off
      settings: SourceProductName=Simulink
  cfblk5 : simulink/Discrete/Transfer Fcn Real Zero  ZeroZ=0.75  ICPrevInput=0.0  DoSatur=off
      settings: SourceProductName=Simulink  SourceProductBaseCode=SL
  cfblk6 : Delay  ShowEnablePort=on
      settings: InputPortMap=u0,e6
  cfblk7 : simulink/Discrete/Transfer Fcn First Order  PoleZ=0.95  ICPrevOutput=0.0  DoSatur=off
      settings: SourceProductName=Simulink
  cfblk8 : simulink/Discrete/Transfer Fcn Real Zero  ZeroZ=0.75  ICPrevInput=0.0  DoSatur=off
      settings: SourceProductName=Simulink  SourceProductBaseCode=SL
  cyemi_{104..110} (7 alike) : DataTypeConversion  OutDataTypeStr=double
  cfblk2 : Outport
  cfblk11 : Outport  Port=2
  cfblk12 : Outport  Port=3
  wires:
  cfblk1/1 -> cfblk11/1
  cfblk10/1 -> cfblk2/1
  cfblk8/1 -> cfblk12/1
  cyemi_104/1 -> cfblk3/1
  cfblk6/1 -> cyemi_104/1
  cyemi_105/1 -> cfblk4/1
  cfblk3/1 -> cyemi_105/1
  cyemi_106/1 -> cfblk5/1
  cfblk4/1 -> cyemi_106/1
  cyemi_107/1 -> cfblk6/1
  cfblk9/1 -> cyemi_107/1, cyemi_108/1
  cyemi_108/1 -> cfblk6/2
  cyemi_109/1 -> cfblk7/1
  cfblk5/1 -> cyemi_109/1
  cyemi_110/1 -> cfblk8/1
  cfblk7/1 -> cyemi_110/1

== system sampleModel2438_pp/cfblk234/cfblk16 ==
  cfblk1 : Inport
  cfblk11 : Inport  Port=2
  cfblk12 : Inport  Port=3
  cfblk13 : Inport  Port=4
  Action Port : ActionPort  ActionType=then
  cfblk10 : simulink/Discrete/Tapped Delay  vinit=0.0  samptime=-1  NumDelays=1  DelayOrder=Oldest  includeCurrent=off
  cfblk3 : DiscreteFir
  cfblk4 : DiscreteIntegrator  SampleTime=-1  ICPrevOutput=DiscIntNeverNeededParam  ICPrevScaledInput=DiscIntNeverNeededParam
  cfblk5 : Delay
  cfblk6 : Delay  ShowEnablePort=on
      settings: InputPortMap=u0,e6
  cfblk7 : DiscreteStateSpace  SampleTime=-1
  cfblk8 : DiscreteFilter
  cfblk9 : simulink/Continuous/PID Controller (2DOF)  Controller=PID  TimeDomain=Discrete-time  SampleTime=-1  IntegratorMethod=Forward Euler  FilterMethod=Forward Euler  Form=Parallel  UseFilter=on  ControllerParametersSource=internal  P=1  I=1  D=0  N=100  b=1  c=1  InitialConditionSource=internal  InitialConditionForIntegrator=0  InitialConditionForFilter=0  ExternalReset=none  LimitOutput=off  UpperSaturationLimit=inf  LowerSaturationLimit=-inf  LinearizeAsGain=off  AntiWindupMode=none  Kb=1  TrackingMode=off  Kt=1  PParamMin=[]  PParamMax=[]  IParamMin=[]  IParamMax=[]  DParamMin=[]  DParamMax=[]  NParamMin=[]  NParamMax=[]  bParamMin=[]  bParamMax=[]  cParamMin=[]  cParamMax=[]  KbParamMin=[]  KbParamMax=[]  KtParamMin=[]  KtParamMax=[]  POutMin=[]  POutMax=[]  IOutMin=[]  IOutMax=[]  DOutMin=[]  DOutMax=[]  NOutMin=[]  NOutMax=[]  bOutMin=[]  bOutMax=[]  cOutMin=[]  cOutMax=[]  KbOutMin=[]  KbOutMax=[]  KtOutMin=[]  KtOutMax=[]  IntegratorOutMin=[]  IntegratorOutMax=[]  FilterOutMin=[]  FilterOutMax=[]  SumOutMin=[]  SumOutMax=[]  Sum1OutMin=[]  Sum1OutMax=[]  Sum2OutMin=[]  Sum2OutMax=[]  Sum3OutMin=[]  Sum3OutMax=[]  SumI1OutMin=[]  SumI1OutMax=[]  SumI2OutMin=[]  SumI2OutMax=[]  SumI3OutMin=[]  SumI3OutMax=[]  SumDOutMin=[]  SumDOutMax=[]  SaturationOutMin=[]  SaturationOutMax=[]  IntegratorContinuousStateAttributes=''  IntegratorStateMustResolveToSignalObject=off  IntegratorRTWStateStorageClass=Auto  FilterContinuousStateAttributes=''  FilterStateMustResolveToSignalObject=off  FilterRTWStateStorageClass=Auto  DifferentiatorICPrevScaledInput=0  DifferentiatorOutMin=[]  DifferentiatorOutMax=[]  FilterDiffOutCoefMin=[]  FilterDiffOutCoefMax=[]  SumDenOutMin=[]  SumDenOutMax=[]  SumNumOutMin=[]  SumNumOutMax=[]  ReciprocalOutMin=[]  ReciprocalOutMax=[]  DivideOutMin=[]  DivideOutMax=[]  TunerSelectOption=Transfer Function Based (PID Tuner App)
  cyemi_{138..147} (10 alike) : DataTypeConversion  OutDataTypeStr=double
  cfblk2 : Outport
  cfblk14 : Outport  Port=2
  wires:
  cfblk13/1 -> cfblk14/1
  cfblk9/1 -> cfblk2/1
  cfblk7/1 -> cyemi_143/1, cyemi_146/1
  cyemi_138/1 -> cfblk10/1
  cfblk5/1 -> cyemi_138/1
  cyemi_139/1 -> cfblk3/1
  cfblk1/1 -> cyemi_139/1
  cyemi_140/1 -> cfblk4/1
  cfblk12/1 -> cyemi_140/1
  cyemi_141/1 -> cfblk5/1
  cfblk3/1 -> cyemi_141/1
  cyemi_142/1 -> cfblk6/1
  cfblk11/1 -> cyemi_142/1
  cyemi_143/1 -> cfblk6/2
  cyemi_144/1 -> cfblk7/1
  cfblk10/1 -> cyemi_144/1
  cyemi_145/1 -> cfblk8/1
  cfblk4/1 -> cyemi_145/1
  cyemi_146/1 -> cfblk9/1
  cyemi_147/1 -> cfblk9/2
  cfblk8/1 -> cyemi_147/1

== system sampleModel2438_pp/cfblk234/cfblk17 ==
  cfblk1 : Inport
  cfblk9 : Inport  Port=2
  cfblk10 : Inport  Port=3
  cfblk11 : Inport  Port=4
  cfblk12 : Inport  Port=5
  Action Port : ActionPort  ActionType=else
  cfblk3 : DiscreteFilter
  cfblk4 : DiscreteTransferFcn
  cfblk5 : UnitDelay  SampleTime=-1
  cfblk6 : DiscreteStateSpace  SampleTime=-1
  cfblk7 : simulink/Discrete/Tapped Delay  vinit=0.0  samptime=-1  NumDelays=1  DelayOrder=Oldest  includeCurrent=off
  cfblk8 : simulink/Discrete/Transfer Fcn Lead or Lag  PoleZ=0.95  ZeroZ=0.75  ICPrevOutput=0.0  ICPrevInput=0.0  DoSatur=off
      settings: SourceProductName=Simulink  SourceProductBaseCode=SL
  cyemi_{153..158} (6 alike) : DataTypeConversion  OutDataTypeStr=double
  cfblk2 : Outport
  wires:
  cfblk8/1 -> cfblk2/1
  cyemi_153/1 -> cfblk3/1
  cfblk7/1 -> cyemi_153/1
  cyemi_154/1 -> cfblk4/1
  cfblk6/1 -> cyemi_154/1
  cyemi_155/1 -> cfblk5/1
  cfblk11/1 -> cyemi_155/1
  cyemi_156/1 -> cfblk6/1
  cfblk3/1 -> cyemi_156/1
  cyemi_157/1 -> cfblk7/1
  cfblk1/1 -> cyemi_157/1
  cyemi_158/1 -> cfblk8/1
  cfblk4/1 -> cyemi_158/1

== system sampleModel2438_pp/cfblk235/cfblk13 ==
  cfblk1 : Inport
  cfblk10 : Inport  Port=2
  Action Port : ActionPort  ActionType=then
  cfblk3 : simulink/Discrete/Transfer Fcn Real Zero  ZeroZ=0.75  ICPrevInput=0.0  DoSatur=off
      settings: SourceProductName=Simulink  SourceProductBaseCode=SL
  cfblk4 : simulink/Continuous/PID Controller  Controller=PID  TimeDomain=Discrete-time  SampleTime=-1  IntegratorMethod=Forward Euler  FilterMethod=Forward Euler  Form=Parallel  UseFilter=on  ControllerParametersSource=internal  P=1  I=1  D=0  N=100  InitialConditionSource=internal  InitialConditionForIntegrator=0  InitialConditionForFilter=0  ExternalReset=none  LimitOutput=off  UpperSaturationLimit=inf  LowerSaturationLimit=-inf  LinearizeAsGain=off  AntiWindupMode=none  Kb=1  TrackingMode=off  Kt=1  PParamMin=[]  PParamMax=[]  IParamMin=[]  IParamMax=[]  DParamMin=[]  DParamMax=[]  NParamMin=[]  NParamMax=[]  KbParamMin=[]  KbParamMax=[]  KtParamMin=[]  KtParamMax=[]  POutMin=[]  POutMax=[]  IOutMin=[]  IOutMax=[]  DOutMin=[]  DOutMax=[]  NOutMin=[]  NOutMax=[]  KbOutMin=[]  KbOutMax=[]  KtOutMin=[]  KtOutMax=[]  IntegratorOutMin=[]  IntegratorOutMax=[]  FilterOutMin=[]  FilterOutMax=[]  SumOutMin=[]  SumOutMax=[]  SumI1OutMin=[]  SumI1OutMax=[]  SumI2OutMin=[]  SumI2OutMax=[]  SumI3OutMin=[]  SumI3OutMax=[]  SumDOutMin=[]  SumDOutMax=[]  SaturationOutMin=[]  SaturationOutMax=[]  IntegratorContinuousStateAttributes=''  IntegratorStateMustResolveToSignalObject=off  IntegratorRTWStateStorageClass=Auto  FilterContinuousStateAttributes=''  FilterStateMustResolveToSignalObject=off  FilterRTWStateStorageClass=Auto  DifferentiatorICPrevScaledInput=0  DifferentiatorOutMin=[]  DifferentiatorOutMax=[]  FilterDiffOutCoefMin=[]  FilterDiffOutCoefMax=[]  SumDenOutMin=[]  SumDenOutMax=[]  SumNumOutMin=[]  SumNumOutMax=[]  ReciprocalOutMin=[]  ReciprocalOutMax=[]  DivideOutMin=[]  DivideOutMax=[]  TunerSelectOption=Transfer Function Based (PID Tuner App)
  cfblk5 : DiscreteStateSpace  SampleTime=-1
  cfblk6 : simulink/Discrete/Transfer Fcn Real Zero  ZeroZ=0.75  ICPrevInput=0.0  DoSatur=off
      settings: SourceProductName=Simulink  SourceProductBaseCode=SL
  cfblk7 : simulink/Discrete/Tapped Delay  vinit=0.0  samptime=-1  NumDelays=1  DelayOrder=Oldest  includeCurrent=off
  cfblk8 : simulink/Discrete/Transfer Fcn Real Zero  ZeroZ=0.75  ICPrevInput=0.0  DoSatur=off
      settings: SourceProductName=Simulink  SourceProductBaseCode=SL
  cfblk9 : simulink/Discrete/Difference  ICPrevInput=0.0  OutMin=[]  OutMax=[]  OutDataTypeStr=Inherit: Inherit via back propagation  OutDataType=fixdt(1, 16)  OutScaling=2^-10  DoSatur=off
  cyemi_{180..186} (7 alike) : DataTypeConversion  OutDataTypeStr=double
  cfblk2 : Outport
  wires:
  cfblk8/1 -> cfblk2/1
  cyemi_180/1 -> cfblk3/1
  cfblk6/1 -> cyemi_180/1
  cyemi_181/1 -> cfblk4/1
  cfblk9/1 -> cyemi_181/1
  cyemi_182/1 -> cfblk5/1
  cfblk1/1 -> cyemi_182/1
  cyemi_183/1 -> cfblk6/1
  cfblk4/1 -> cyemi_183/1
  cyemi_184/1 -> cfblk7/1
  cfblk5/1 -> cyemi_184/1
  cyemi_185/1 -> cfblk8/1
  cfblk10/1 -> cyemi_185/1
  cyemi_186/1 -> cfblk9/1
  cfblk7/1 -> cyemi_186/1

== system sampleModel2438_pp/cfblk235/cfblk14 ==
  cfblk1 : Inport
  cfblk12 : Inport  Port=2
  Action Port : ActionPort  ActionType=else
  cfblk10 : UnitDelay  SampleTime=-1
  cfblk11 : simulink/Continuous/PID Controller  Controller=PID  TimeDomain=Discrete-time  SampleTime=-1  IntegratorMethod=Forward Euler  FilterMethod=Forward Euler  Form=Parallel  UseFilter=on  ControllerParametersSource=internal  P=1  I=1  D=0  N=100  InitialConditionSource=internal  InitialConditionForIntegrator=0  InitialConditionForFilter=0  ExternalReset=none  LimitOutput=off  UpperSaturationLimit=inf  LowerSaturationLimit=-inf  LinearizeAsGain=off  AntiWindupMode=none  Kb=1  TrackingMode=off  Kt=1  PParamMin=[]  PParamMax=[]  IParamMin=[]  IParamMax=[]  DParamMin=[]  DParamMax=[]  NParamMin=[]  NParamMax=[]  KbParamMin=[]  KbParamMax=[]  KtParamMin=[]  KtParamMax=[]  POutMin=[]  POutMax=[]  IOutMin=[]  IOutMax=[]  DOutMin=[]  DOutMax=[]  NOutMin=[]  NOutMax=[]  KbOutMin=[]  KbOutMax=[]  KtOutMin=[]  KtOutMax=[]  IntegratorOutMin=[]  IntegratorOutMax=[]  FilterOutMin=[]  FilterOutMax=[]  SumOutMin=[]  SumOutMax=[]  SumI1OutMin=[]  SumI1OutMax=[]  SumI2OutMin=[]  SumI2OutMax=[]  SumI3OutMin=[]  SumI3OutMax=[]  SumDOutMin=[]  SumDOutMax=[]  SaturationOutMin=[]  SaturationOutMax=[]  IntegratorContinuousStateAttributes=''  IntegratorStateMustResolveToSignalObject=off  IntegratorRTWStateStorageClass=Auto  FilterContinuousStateAttributes=''  FilterStateMustResolveToSignalObject=off  FilterRTWStateStorageClass=Auto  DifferentiatorICPrevScaledInput=0  DifferentiatorOutMin=[]  DifferentiatorOutMax=[]  FilterDiffOutCoefMin=[]  FilterDiffOutCoefMax=[]  SumDenOutMin=[]  SumDenOutMax=[]  SumNumOutMin=[]  SumNumOutMax=[]  ReciprocalOutMin=[]  ReciprocalOutMax=[]  DivideOutMin=[]  DivideOutMax=[]  TunerSelectOption=Transfer Function Based (PID Tuner App)
  cfblk15 : Delay
  cfblk16 : Delay
  cfblk3 : DiscreteFir
  cfblk4 : simulink/Discrete/Difference  ICPrevInput=0.0  OutMin=[]  OutMax=[]  OutDataTypeStr=Inherit: Inherit via back propagation  OutDataType=fixdt(1, 16)  OutScaling=2^-10  DoSatur=off
  cfblk5 : DiscreteTransferFcn
  cfblk6 : simulink/Discrete/Tapped Delay  vinit=0.0  samptime=-1  NumDelays=1  DelayOrder=Oldest  includeCurrent=off
  cfblk7 : simulink/Discrete/Transfer Fcn Lead or Lag  PoleZ=0.95  ZeroZ=0.75  ICPrevOutput=0.0  ICPrevInput=0.0  DoSatur=off
      settings: SourceProductName=Simulink  SourceProductBaseCode=SL
  cfblk8 : simulink/Continuous/PID Controller (2DOF)  Controller=PID  TimeDomain=Discrete-time  SampleTime=-1  IntegratorMethod=Forward Euler  FilterMethod=Forward Euler  Form=Parallel  UseFilter=on  ControllerParametersSource=internal  P=1  I=1  D=0  N=100  b=1  c=1  InitialConditionSource=internal  InitialConditionForIntegrator=0  InitialConditionForFilter=0  ExternalReset=none  LimitOutput=off  UpperSaturationLimit=inf  LowerSaturationLimit=-inf  LinearizeAsGain=off  AntiWindupMode=none  Kb=1  TrackingMode=off  Kt=1  PParamMin=[]  PParamMax=[]  IParamMin=[]  IParamMax=[]  DParamMin=[]  DParamMax=[]  NParamMin=[]  NParamMax=[]  bParamMin=[]  bParamMax=[]  cParamMin=[]  cParamMax=[]  KbParamMin=[]  KbParamMax=[]  KtParamMin=[]  KtParamMax=[]  POutMin=[]  POutMax=[]  IOutMin=[]  IOutMax=[]  DOutMin=[]  DOutMax=[]  NOutMin=[]  NOutMax=[]  bOutMin=[]  bOutMax=[]  cOutMin=[]  cOutMax=[]  KbOutMin=[]  KbOutMax=[]  KtOutMin=[]  KtOutMax=[]  IntegratorOutMin=[]  IntegratorOutMax=[]  FilterOutMin=[]  FilterOutMax=[]  SumOutMin=[]  SumOutMax=[]  Sum1OutMin=[]  Sum1OutMax=[]  Sum2OutMin=[]  Sum2OutMax=[]  Sum3OutMin=[]  Sum3OutMax=[]  SumI1OutMin=[]  SumI1OutMax=[]  SumI2OutMin=[]  SumI2OutMax=[]  SumI3OutMin=[]  SumI3OutMax=[]  SumDOutMin=[]  SumDOutMax=[]  SaturationOutMin=[]  SaturationOutMax=[]  IntegratorContinuousStateAttributes=''  IntegratorStateMustResolveToSignalObject=off  IntegratorRTWStateStorageClass=Auto  FilterContinuousStateAttributes=''  FilterStateMustResolveToSignalObject=off  FilterRTWStateStorageClass=Auto  DifferentiatorICPrevScaledInput=0  DifferentiatorOutMin=[]  DifferentiatorOutMax=[]  FilterDiffOutCoefMin=[]  FilterDiffOutCoefMax=[]  SumDenOutMin=[]  SumDenOutMax=[]  SumNumOutMin=[]  SumNumOutMax=[]  ReciprocalOutMin=[]  ReciprocalOutMax=[]  DivideOutMin=[]  DivideOutMax=[]  TunerSelectOption=Transfer Function Based (PID Tuner App)
  cfblk9 : DiscreteStateSpace  SampleTime=-1
  cyemi_{189..200} (12 alike) : DataTypeConversion  OutDataTypeStr=double
  cfblk2 : Outport
  cfblk13 : Outport  Port=2
  cfblk14 : Outport  Port=3
  wires:
  cfblk9/1 -> cyemi_190/1, cyemi_199/1
  cfblk12/1 -> cfblk13/1
  cfblk7/1 -> cfblk2/1
  cfblk3/1 -> cfblk14/1
  cfblk6/1 -> cyemi_192/1, cyemi_193/1
  cyemi_189/1 -> cfblk10/1
  cfblk11/1 -> cyemi_189/1
  cyemi_190/1 -> cfblk11/1
  cyemi_191/1 -> cfblk15/1
  cfblk10/1 -> cyemi_191/1
  cyemi_192/1 -> cfblk16/1
  cyemi_193/1 -> cfblk3/1
  cyemi_194/1 -> cfblk4/1
  cfblk1/1 -> cyemi_194/1
  cyemi_195/1 -> cfblk5/1
  cfblk15/1 -> cyemi_195/1
  cyemi_196/1 -> cfblk6/1
  cfblk8/1 -> cyemi_196/1
  cyemi_197/1 -> cfblk7/1
  cfblk4/1 -> cyemi_197/1
  cyemi_198/1 -> cfblk8/1
  cfblk16/1 -> cyemi_198/1
  cyemi_199/1 -> cfblk8/2
  cyemi_200/1 -> cfblk9/1
  cfblk5/1 -> cyemi_200/1

== system sampleModel2438_pp/cfblk239/cfblk17 ==
  cfblk1 : Inport
  cfblk9 : Inport  Port=2
  cfblk10 : Inport  Port=3
  Action Port : ActionPort  ActionType=then
  cfblk3 : DiscreteIntegrator  SampleTime=-1  ICPrevOutput=DiscIntNeverNeededParam  ICPrevScaledInput=DiscIntNeverNeededParam
  cfblk4 : simulink/Discrete/Transfer Fcn Real Zero  ZeroZ=0.75  ICPrevInput=0.0  DoSatur=off
      settings: SourceProductName=Simulink  SourceProductBaseCode=SL
  cfblk5 : simulink/Discrete/Transfer Fcn Lead or Lag  PoleZ=0.95  ZeroZ=0.75  ICPrevOutput=0.0  ICPrevInput=0.0  DoSatur=off
      settings: SourceProductName=Simulink  SourceProductBaseCode=SL
  cfblk6 : DiscreteStateSpace  SampleTime=-1
  cfblk7 : simulink/Discrete/Transfer Fcn Lead or Lag  PoleZ=0.95  ZeroZ=0.75  ICPrevOutput=0.0  ICPrevInput=0.0  DoSatur=off
      settings: SourceProductName=Simulink  SourceProductBaseCode=SL
  cfblk8 : UnitDelay  SampleTime=-1
  cyemi_{259..264} (6 alike) : DataTypeConversion  OutDataTypeStr=double
  cfblk2 : Outport
  cfblk11 : Outport  Port=2
  cfblk12 : Outport  Port=3
  cfblk13 : Outport  Port=4
  wires:
  cfblk8/1 -> cfblk2/1
  cfblk10/1 -> cyemi_259/1, cyemi_263/1
  cfblk5/1 -> cfblk11/1
  cfblk3/1 -> cfblk12/1
  cfblk7/1 -> cfblk13/1
  cyemi_259/1 -> cfblk3/1
  cyemi_260/1 -> cfblk4/1
  cfblk1/1 -> cyemi_260/1
  cyemi_261/1 -> cfblk5/1
  cfblk6/1 -> cyemi_261/1
  cyemi_262/1 -> cfblk6/1
  cfblk9/1 -> cyemi_262/1
  cyemi_263/1 -> cfblk7/1
  cyemi_264/1 -> cfblk8/1
  cfblk4/1 -> cyemi_264/1

== system sampleModel2438_pp/cfblk239/cfblk18 ==
  cfblk1 : Inport
  cfblk13 : Inport  Port=2
  cfblk14 : Inport  Port=3
  Action Port : ActionPort  ActionType=else
  cfblk{4,7,10,18} (4 alike) : Delay
  cfblk11 : UnitDelay  SampleTime=-1
  cfblk12 : DiscreteStateSpace  SampleTime=-1
  cfblk{3,5,8..9} (4 alike) : simulink/Discrete/Tapped Delay  vinit=0.0  samptime=-1  NumDelays=1  DelayOrder=Oldest  includeCurrent=off
  cfblk6 : DiscreteZeroPole  Poles=[0 0.5]  Gain=1  SampleTime=-1
  cyemi_{268..278} (11 alike) : DataTypeConversion  OutDataTypeStr=double
  cfblk2 : Outport
  cfblk15 : Outport  Port=2
  cfblk16 : Outport  Port=3
  cfblk17 : Outport  Port=4
  wires:
  cfblk10/1 -> cfblk17/1
  cfblk7/1 -> cfblk2/1
  cfblk14/1 -> cfblk16/1
  cfblk11/1 -> cfblk15/1, cyemi_273/1
  cyemi_268/1 -> cfblk10/1
  cfblk4/1 -> cyemi_268/1
  cyemi_269/1 -> cfblk11/1
  cfblk9/1 -> cyemi_269/1
  cyemi_270/1 -> cfblk12/1
  cfblk13/1 -> cyemi_270/1
  cyemi_271/1 -> cfblk18/1
  cfblk6/1 -> cyemi_271/1
  cyemi_272/1 -> cfblk3/1
  cfblk18/1 -> cyemi_272/1
  cyemi_273/1 -> cfblk4/1
  cyemi_274/1 -> cfblk5/1
  cfblk3/1 -> cyemi_274/1
  cyemi_275/1 -> cfblk6/1
  cfblk8/1 -> cyemi_275/1
  cyemi_276/1 -> cfblk7/1
  cfblk1/1 -> cyemi_276/1
  cyemi_277/1 -> cfblk8/1
  cfblk5/1 -> cyemi_277/1
  cyemi_278/1 -> cfblk9/1
  cfblk12/1 -> cyemi_278/1
